simulink model "Dinamica_numerica_MPC"  (R2024b)
(part 3 of 4)

% A_drag(4,4) = (B_c*mu*rho*(cos(u_c - atan2(e_yc, e_xc) + (13*sin(3*u_c - 3*atan2(e_yc, e_xc))*(e_xc^2 + e_yc^2)^(3/2))/12 + sin(u_c - atan2(e_yc, e_xc))*(2*(e_xc^2 + e_yc^2)^(1/2) - (e_xc^2 + e_yc^2)^(3/2)/4) + sin(2*u_c - 2*atan2(e_yc, e_xc))*((5*e_xc^2)/4 + (5*e_yc^2)/4)) + (e_xc^2 + e_yc^2)^(1/2))*(delta_B + 1)*(2*cos(u_c - atan2(e_yc, e_xc) + (13*sin(3*u_c - 3*atan2(e_yc, e_xc))*(e_xc^2 + e_yc^2)^(3/2))/12 + sin(u_c - atan2(e_yc, e_xc))*(2*(e_xc^2 + e_yc^2)^(1/2) - (e_xc^2 + e_yc^2)^(3/2)/4) + sin(2*u_c - 2*atan2(e_yc, e_xc))*((5*e_xc^2)/4 + (5*e_yc^2)/4))*(e_xc^2 + e_yc^2)^(1/2) + e_xc^2 + e_yc^2 + 1)^(1/2))/(a_c*(e_xc^2 + e_yc^2)^(1/2)*(-mu/(a_c*(e_xc^2 + e_yc^2 - 1)))^(1/2)*(e_xc^2 + e_yc^2 - 1)) - (2*B_c*e_yc^2*mu*rho*(cos(u_c - atan2(e_yc, e_xc) + (13*sin(3*u_c - 3*atan2(e_yc, e_xc))*(e_xc^2 + e_yc^2)^(3/2))/12 + sin(u_c - atan2(e_yc, e_xc))*(2*(e_xc^2 + e_yc^2)^(1/2) - (e_xc^2 + e_yc^2)^(3/2)/4) + sin(2*u_c - 2*atan2(e_yc, e_xc))*((5*e_xc^2)/4 + (5*e_yc^2)/4)) + (e_xc^2 + e_yc^2)^(1/2))*(delta_B + 1)*(2*cos(u_c - atan2(e_yc, e_xc) + (13*sin(3*u_c - 3*atan2(e_yc, e_xc))*(e_xc^2 + e_yc^2)^(3/2))/12 + sin(u_c - atan2(e_yc, e_xc))*(2*(e_xc^2 + e_yc^2)^(1/2) - (e_xc^2 + e_yc^2)^(3/2)/4) + sin(2*u_c - 2*atan2(e_yc, e_xc))*((5*e_xc^2)/4 + (5*e_yc^2)/4))*(e_xc^2 + e_yc^2)^(1/2) + e_xc^2 + e_yc^2 + 1)^(1/2))/(a_c*(e_xc^2 + e_yc^2)^(1/2)*(-mu/(a_c*(e_xc^2 + e_yc^2 - 1)))^(1/2)*(e_xc^2 + e_yc^2 - 1)^2) - (B_c*e_yc^2*mu*rho*(cos(u_c - atan2(e_yc, e_xc) + (13*sin(3*u_c - 3*atan2(e_yc, e_xc))*(e_xc^2 + e_yc^2)^(3/2))/12 + sin(u_c - atan2(e_yc, e_xc))*(2*(e_xc^2 + e_yc^2)^(1/2) - (e_xc^2 + e_yc^2)^(3/2)/4) + sin(2*u_c - 2*atan2(e_yc, e_xc))*((5*e_xc^2)/4 + (5*e_yc^2)/4)) + (e_xc^2 + e_yc^2)^(1/2))*(delta_B + 1)*(2*cos(u_c - atan2(e_yc, e_xc) + (13*sin(3*u_c - 3*atan2(e_yc, e_xc))*(e_xc^2 + e_yc^2)^(3/2))/12 + sin(u_c - atan2(e_yc, e_xc))*(2*(e_xc^2 + e_yc^2)^(1/2) - (e_xc^2 + e_yc^2)^(3/2)/4) + sin(2*u_c - 2*atan2(e_yc, e_xc))*((5*e_xc^2)/4 + (5*e_yc^2)/4))*(e_xc^2 + e_yc^2)^(1/2) + e_xc^2 + e_yc^2 + 1)^(1/2))/(a_c*(e_xc^2 + e_yc^2)^(3/2)*(-mu/(a_c*(e_xc^2 + e_yc^2 - 1)))^(1/2)*(e_xc^2 + e_yc^2 - 1)) + (B_c*e_yc*mu*rho*(delta_B + 1)*(e_yc/(e_xc^2 + e_yc^2)^(1/2) + sin(u_c - atan2(e_yc, e_xc) + (13*sin(3*u_c - 3*atan2(e_yc, e_xc))*(e_xc^2 + e_yc^2)^(3/2))/12 + sin(u_c - atan2(e_yc, e_xc))*(2*(e_xc^2 + e_yc^2)^(1/2) - (e_xc^2 + e_yc^2)^(3/2)/4) + sin(2*u_c - 2*atan2(e_yc, e_xc))*((5*e_xc^2)/4 + (5*e_yc^2)/4))*(e_xc/(e_xc^2 + e_yc^2) - sin(u_c - atan2(e_yc, e_xc))*((2*e_yc)/(e_xc^2 + e_yc^2)^(1/2) - (3*e_yc*(e_xc^2 + e_yc^2)^(1/2))/4) - (5*e_yc*sin(2*u_c - 2*atan2(e_yc, e_xc)))/2 + (13*e_xc*cos(3*u_c - 3*atan2(e_yc, e_xc))*(e_xc^2 + e_yc^2)^(1/2))/4 - (13*e_yc*sin(3*u_c - 3*atan2(e_yc, e_xc))*(e_xc^2 + e_yc^2)^(1/2))/4 + (e_xc*cos(u_c - atan2(e_yc, e_xc))*(2*(e_xc^2 + e_yc^2)^(1/2) - (e_xc^2 + e_yc^2)^(3/2)/4))/(e_xc^2 + e_yc^2) + (2*e_xc*cos(2*u_c - 2*atan2(e_yc, e_xc))*((5*e_xc^2)/4 + (5*e_yc^2)/4))/(e_xc^2 + e_yc^2)))*(2*cos(u_c - atan2(e_yc, e_xc) + (13*sin(3*u_c - 3*atan2(e_yc, e_xc))*(e_xc^2 + e_yc^2)^(3/2))/12 + sin(u_c - atan2(e_yc, e_xc))*(2*(e_xc^2 + e_yc^2)^(1/2) - (e_xc^2 + e_yc^2)^(3/2)/4) + sin(2*u_c - 2*atan2(e_yc, e_xc))*((5*e_xc^2)/4 + (5*e_yc^2)/4))*(e_xc^2 + e_yc^2)^(1/2) + e_xc^2 + e_yc^2 + 1)^(1/2))/(a_c*(e_xc^2 + e_yc^2)^(1/2)*(-mu/(a_c*(e_xc^2 + e_yc^2 - 1)))^(1/2)*(e_xc^2 + e_yc^2 - 1)) - (B_c*e_yc^2*mu^2*rho*(cos(u_c - atan2(e_yc, e_xc) + (13*sin(3*u_c - 3*atan2(e_yc, e_xc))*(e_xc^2 + e_yc^2)^(3/2))/12 + sin(u_c - atan2(e_yc, e_xc))*(2*(e_xc^2 + e_yc^2)^(1/2) - (e_xc^2 + e_yc^2)^(3/2)/4) + sin(2*u_c - 2*atan2(e_yc, e_xc))*((5*e_xc^2)/4 + (5*e_yc^2)/4)) + (e_xc^2 + e_yc^2)^(1/2))*(delta_B + 1)*(2*cos(u_c - atan2(e_yc, e_xc) + (13*sin(3*u_c - 3*atan2(e_yc, e_xc))*(e_xc^2 + e_yc^2)^(3/2))/12 + sin(u_c - atan2(e_yc, e_xc))*(2*(e_xc^2 + e_yc^2)^(1/2) - (e_xc^2 + e_yc^2)^(3/2)/4) + sin(2*u_c - 2*atan2(e_yc, e_xc))*((5*e_xc^2)/4 + (5*e_yc^2)/4))*(e_xc^2 + e_yc^2)^(1/2) + e_xc^2 + e_yc^2 + 1)^(1/2))/(a_c^2*(e_xc^2 + e_yc^2)^(1/2)*(-mu/(a_c*(e_xc^2 + e_yc^2 - 1)))^(3/2)*(e_xc^2 + e_yc^2 - 1)^3) - (2*B_c*e_xc*e_yc*mu*rho*sin(u_c - atan2(e_yc, e_xc) + (13*sin(3*u_c - 3*atan2(e_yc, e_xc))*(e_xc^2 + e_yc^2)^(3/2))/12 + sin(u_c - atan2(e_yc, e_xc))*(2*(e_xc^2 + e_yc^2)^(1/2) - (e_xc^2 + e_yc^2)^(3/2)/4) + sin(2*u_c - 2*atan2(e_yc, e_xc))*((5*e_xc^2)/4 + (5*e_yc^2)/4))*(delta_B + 1)*(2*cos(u_c - atan2(e_yc, e_xc) + (13*sin(3*u_c - 3*atan2(e_yc, e_xc))*(e_xc^2 + e_yc^2)^(3/2))/12 + sin(u_c - atan2(e_yc, e_xc))*(2*(e_xc^2 + e_yc^2)^(1/2) - (e_xc^2 + e_yc^2)^(3/2)/4) + sin(2*u_c - 2*atan2(e_yc, e_xc))*((5*e_xc^2)/4 + (5*e_yc^2)/4))*(e_xc^2 + e_yc^2)^(1/2) + e_xc^2 + e_yc^2 + 1)^(1/2))/(a_c*(e_xc^2 + e_yc^2)^(1/2)*(-mu/(a_c*(e_xc^2 + e_yc^2 - 1)))^(1/2)*(e_xc^2 + e_yc^2 - 1)^2) - (B_c*e_xc*e_yc*mu*rho*sin(u_c - atan2(e_yc, e_xc) + (13*sin(3*u_c - 3*atan2(e_yc, e_xc))*(e_xc^2 + e_yc^2)^(3/2))/12 + sin(u_c - atan2(e_yc, e_xc))*(2*(e_xc^2 + e_yc^2)^(1/2) - (e_xc^2 + e_yc^2)^(3/2)/4) + sin(2*u_c - 2*atan2(e_yc, e_xc))*((5*e_xc^2)/4 + (5*e_yc^2)/4))*(delta_B + 1)*(2*cos(u_c - atan2(e_yc, e_xc) + (13*sin(3*u_c - 3*atan2(e_yc, e_xc))*(e_xc^2 + e_yc^2)^(3/2))/12 + sin(u_c - atan2(e_yc, e_xc))*(2*(e_xc^2 + e_yc^2)^(1/2) - (e_xc^2 + e_yc^2)^(3/2)/4) + sin(2*u_c - 2*atan2(e_yc, e_xc))*((5*e_xc^2)/4 + (5*e_yc^2)/4))*(e_xc^2 + e_yc^2)^(1/2) + e_xc^2 + e_yc^2 + 1)^(1/2))/(a_c*(e_xc^2 + e_yc^2)^(3/2)*(-mu/(a_c*(e_xc^2 + e_yc^2 - 1)))^(1/2)*(e_xc^2 + e_yc^2 - 1)) + (B_c*e_xc*mu*rho*sin(u_c - atan2(e_yc, e_xc) + (13*sin(3*u_c - 3*atan2(e_yc, e_xc))*(e_xc^2 + e_yc^2)^(3/2))/12 + sin(u_c - atan2(e_yc, e_xc))*(2*(e_xc^2 + e_yc^2)^(1/2) - (e_xc^2 + e_yc^2)^(3/2)/4) + sin(2*u_c - 2*atan2(e_yc, e_xc))*((5*e_xc^2)/4 + (5*e_yc^2)/4))*(delta_B + 1)*(2*e_yc + (2*e_yc*cos(u_c - atan2(e_yc, e_xc) + (13*sin(3*u_c - 3*atan2(e_yc, e_xc))*(e_xc^2 + e_yc^2)^(3/2))/12 + sin(u_c - atan2(e_yc, e_xc))*(2*(e_xc^2 + e_yc^2)^(1/2) - (e_xc^2 + e_yc^2)^(3/2)/4) + sin(2*u_c - 2*atan2(e_yc, e_xc))*((5*e_xc^2)/4 + (5*e_yc^2)/4)))/(e_xc^2 + e_yc^2)^(1/2) + 2*sin(u_c - atan2(e_yc, e_xc) + (13*sin(3*u_c - 3*atan2(e_yc, e_xc))*(e_xc^2 + e_yc^2)^(3/2))/12 + sin(u_c - atan2(e_yc, e_xc))*(2*(e_xc^2 + e_yc^2)^(1/2) - (e_xc^2 + e_yc^2)^(3/2)/4) + sin(2*u_c - 2*atan2(e_yc, e_xc))*((5*e_xc^2)/4 + (5*e_yc^2)/4))*(e_xc^2 + e_yc^2)^(1/2)*(e_xc/(e_xc^2 + e_yc^2) - sin(u_c - atan2(e_yc, e_xc))*((2*e_yc)/(e_xc^2 + e_yc^2)^(1/2) - (3*e_yc*(e_xc^2 + e_yc^2)^(1/2))/4) - (5*e_yc*sin(2*u_c - 2*atan2(e_yc, e_xc)))/2 + (13*e_xc*cos(3*u_c - 3*atan2(e_yc, e_xc))*(e_xc^2 + e_yc^2)^(1/2))/4 - (13*e_yc*sin(3*u_c - 3*atan2(e_yc, e_xc))*(e_xc^2 + e_yc^2)^(1/2))/4 + (e_xc*cos(u_c - atan2(e_yc, e_xc))*(2*(e_xc^2 + e_yc^2)^(1/2) - (e_xc^2 + e_yc^2)^(3/2)/4))/(e_xc^2 + e_yc^2) + (2*e_xc*cos(2*u_c - 2*atan2(e_yc, e_xc))*((5*e_xc^2)/4 + (5*e_yc^2)/4))/(e_xc^2 + e_yc^2))))/(2*a_c*(e_xc^2 + e_yc^2)^(1/2)*(-mu/(a_c*(e_xc^2 + e_yc^2 - 1)))^(1/2)*(e_xc^2 + e_yc^2 - 1)*(2*cos(u_c - atan2(e_yc, e_xc) + (13*sin(3*u_c - 3*atan2(e_yc, e_xc))*(e_xc^2 + e_yc^2)^(3/2))/12 + sin(u_c - atan2(e_yc, e_xc))*(2*(e_xc^2 + e_yc^2)^(1/2) - (e_xc^2 + e_yc^2)^(3/2)/4) + sin(2*u_c - 2*atan2(e_yc, e_xc))*((5*e_xc^2)/4 + (5*e_yc^2)/4))*(e_xc^2 + e_yc^2)^(1/2) + e_xc^2 + e_yc^2 + 1)^(1/2)) - (B_c*e_xc*e_yc*mu^2*rho*sin(u_c - atan2(e_yc, e_xc) + (13*sin(3*u_c - 3*atan2(e_yc, e_xc))*(e_xc^2 + e_yc^2)^(3/2))/12 + sin(u_c - atan2(e_yc, e_xc))*(2*(e_xc^2 + e_yc^2)^(1/2) - (e_xc^2 + e_yc^2)^(3/2)/4) + sin(2*u_c - 2*atan2(e_yc, e_xc))*((5*e_xc^2)/4 + (5*e_yc^2)/4))*(delta_B + 1)*(2*cos(u_c - atan2(e_yc, e_xc) + (13*sin(3*u_c - 3*atan2(e_yc, e_xc))*(e_xc^2 + e_yc^2)^(3/2))/12 + sin(u_c - atan2(e_yc, e_xc))*(2*(e_xc^2 + e_yc^2)^(1/2) - (e_xc^2 + e_yc^2)^(3/2)/4) + sin(2*u_c - 2*atan2(e_yc, e_xc))*((5*e_xc^2)/4 + (5*e_yc^2)/4))*(e_xc^2 + e_yc^2)^(1/2) + e_xc^2 + e_yc^2 + 1)^(1/2))/(a_c^2*(e_xc^2 + e_yc^2)^(1/2)*(-mu/(a_c*(e_xc^2 + e_yc^2 - 1)))^(3/2)*(e_xc^2 + e_yc^2 - 1)^3) - (B_c*e_xc*mu*rho*cos(u_c - atan2(e_yc, e_xc) + (13*sin(3*u_c - 3*atan2(e_yc, e_xc))*(e_xc^2 + e_yc^2)^(3/2))/12 + sin(u_c - atan2(e_yc, e_xc))*(2*(e_xc^2 + e_yc^2)^(1/2) - (e_xc^2 + e_yc^2)^(3/2)/4) + sin(2*u_c - 2*atan2(e_yc, e_xc))*((5*e_xc^2)/4 + (5*e_yc^2)/4))*(delta_B + 1)*(2*cos(u_c - atan2(e_yc, e_xc) + (13*sin(3*u_c - 3*atan2(e_yc, e_xc))*(e_xc^2 + e_yc^2)^(3/2))/12 + sin(u_c - atan2(e_yc, e_xc))*(2*(e_xc^2 + e_yc^2)^(1/2) - (e_xc^2 + e_yc^2)^(3/2)/4) + sin(2*u_c - 2*atan2(e_yc, e_xc))*((5*e_xc^2)/4 + (5*e_yc^2)/4))*(e_xc^2 + e_yc^2)^(1/2) + e_xc^2 + e_yc^2 + 1)^(1/2)*(e_xc/(e_xc^2 + e_yc^2) - sin(u_c - atan2(e_yc, e_xc))*((2*e_yc)/(e_xc^2 + e_yc^2)^(1/2) - (3*e_yc*(e_xc^2 + e_yc^2)^(1/2))/4) - (5*e_yc*sin(2*u_c - 2*atan2(e_yc, e_xc)))/2 + (13*e_xc*cos(3*u_c - 3*atan2(e_yc, e_xc))*(e_xc^2 + e_yc^2)^(1/2))/4 - (13*e_yc*sin(3*u_c - 3*atan2(e_yc, e_xc))*(e_xc^2 + e_yc^2)^(1/2))/4 + (e_xc*cos(u_c - atan2(e_yc, e_xc))*(2*(e_xc^2 + e_yc^2)^(1/2) - (e_xc^2 + e_yc^2)^(3/2)/4))/(e_xc^2 + e_yc^2) + (2*e_xc*cos(2*u_c - 2*atan2(e_yc, e_xc))*((5*e_xc^2)/4 + (5*e_yc^2)/4))/(e_xc^2 + e_yc^2)))/(a_c*(e_xc^2 + e_yc^2)^(1/2)*(-mu/(a_c*(e_xc^2 + e_yc^2 - 1)))^(1/2)*(e_xc^2 + e_yc^2 - 1)) + (B_c*e_yc*mu*rho*(cos(u_c - atan2(e_yc, e_xc) + (13*sin(3*u_c - 3*atan2(e_yc, e_xc))*(e_xc^2 + e_yc^2)^(3/2))/12 + sin(u_c - atan2(e_yc, e_xc))*(2*(e_xc^2 + e_yc^2)^(1/2) - (e_xc^2 + e_yc^2)^(3/2)/4) + sin(2*u_c - 2*atan2(e_yc, e_xc))*((5*e_xc^2)/4 + (5*e_yc^2)/4)) + (e_xc^2 + e_yc^2)^(1/2))*(delta_B + 1)*(2*e_yc + (2*e_yc*cos(u_c - atan2(e_yc, e_xc) + (13*sin(3*u_c - 3*atan2(e_yc, e_xc))*(e_xc^2 + e_yc^2)^(3/2))/12 + sin(u_c - atan2(e_yc, e_xc))*(2*(e_xc^2 + e_yc^2)^(1/2) - (e_xc^2 + e_yc^2)^(3/2)/4) + sin(2*u_c - 2*atan2(e_yc, e_xc))*((5*e_xc^2)/4 + (5*e_yc^2)/4)))/(e_xc^2 + e_yc^2)^(1/2) + 2*sin(u_c - atan2(e_yc, e_xc) + (13*sin(3*u_c - 3*atan2(e_yc, e_xc))*(e_xc^2 + e_yc^2)^(3/2))/12 + sin(u_c - atan2(e_yc, e_xc))*(2*(e_xc^2 + e_yc^2)^(1/2) - (e_xc^2 + e_yc^2)^(3/2)/4) + sin(2*u_c - 2*atan2(e_yc, e_xc))*((5*e_xc^2)/4 + (5*e_yc^2)/4))*(e_xc^2 + e_yc^2)^(1/2)*(e_xc/(e_xc^2 + e_yc^2) - sin(u_c - atan2(e_yc, e_xc))*((2*e_yc)/(e_xc^2 + e_yc^2)^(1/2) - (3*e_yc*(e_xc^2 + e_yc^2)^(1/2))/4) - (5*e_yc*sin(2*u_c - 2*atan2(e_yc, e_xc)))/2 + (13*e_xc*cos(3*u_c - 3*atan2(e_yc, e_xc))*(e_xc^2 + e_yc^2)^(1/2))/4 - (13*e_yc*sin(3*u_c - 3*atan2(e_yc, e_xc))*(e_xc^2 + e_yc^2)^(1/2))/4 + (e_xc*cos(u_c - atan2(e_yc, e_xc))*(2*(e_xc^2 + e_yc^2)^(1/2) - (e_xc^2 + e_yc^2)^(3/2)/4))/(e_xc^2 + e_yc^2) + (2*e_xc*cos(2*u_c - 2*atan2(e_yc, e_xc))*((5*e_xc^2)/4 + (5*e_yc^2)/4))/(e_xc^2 + e_yc^2))))/(2*a_c*(e_xc^2 + e_yc^2)^(1/2)*(-mu/(a_c*(e_xc^2 + e_yc^2 - 1)))^(1/2)*(e_xc^2 + e_yc^2 - 1)*(2*cos(u_c - atan2(e_yc, e_xc) + (13*sin(3*u_c - 3*atan2(e_yc, e_xc))*(e_xc^2 + e_yc^2)^(3/2))/12 + sin(u_c - atan2(e_yc, e_xc))*(2*(e_xc^2 + e_yc^2)^(1/2) - (e_xc^2 + e_yc^2)^(3/2)/4) + sin(2*u_c - 2*atan2(e_yc, e_xc))*((5*e_xc^2)/4 + (5*e_yc^2)/4))*(e_xc^2 + e_yc^2)^(1/2) + e_xc^2 + e_yc^2 + 1)^(1/2));
% A_drag(4,5) = 0;
% A_drag(4,6) = (B_c*e_xc*mu*rho*sin(u_c - atan2(e_yc, e_xc) + (13*sin(3*u_c - 3*atan2(e_yc, e_xc))*(e_xc^2 + e_yc^2)^(3/2))/12 + sin(u_c - atan2(e_yc, e_xc))*(2*(e_xc^2 + e_yc^2)^(1/2) - (e_xc^2 + e_yc^2)^(3/2)/4) + sin(2*u_c - 2*atan2(e_yc, e_xc))*((5*e_xc^2)/4 + (5*e_yc^2)/4))^2*(delta_B + 1)*(1/tan(i_c) + (2*cos(2*u_c - 2*atan2(e_yc, e_xc))*((5*e_xc^2)/4 + (5*e_yc^2)/4))/tan(i_c) + (13*cos(3*u_c - 3*atan2(e_yc, e_xc))*(e_xc^2 + e_yc^2)^(3/2))/(4*tan(i_c)) + (cos(u_c - atan2(e_yc, e_xc))*(2*(e_xc^2 + e_yc^2)^(1/2) - (e_xc^2 + e_yc^2)^(3/2)/4))/tan(i_c)))/(a_c*(-mu/(a_c*(e_xc^2 + e_yc^2 - 1)))^(1/2)*(e_xc^2 + e_yc^2 - 1)*(2*cos(u_c - atan2(e_yc, e_xc) + (13*sin(3*u_c - 3*atan2(e_yc, e_xc))*(e_xc^2 + e_yc^2)^(3/2))/12 + sin(u_c - atan2(e_yc, e_xc))*(2*(e_xc^2 + e_yc^2)^(1/2) - (e_xc^2 + e_yc^2)^(3/2)/4) + sin(2*u_c - 2*atan2(e_yc, e_xc))*((5*e_xc^2)/4 + (5*e_yc^2)/4))*(e_xc^2 + e_yc^2)^(1/2) + e_xc^2 + e_yc^2 + 1)^(1/2)) + (B_c*e_yc*mu*rho*sin(u_c - atan2(e_yc, e_xc) + (13*sin(3*u_c - 3*atan2(e_yc, e_xc))*(e_xc^2 + e_yc^2)^(3/2))/12 + sin(u_c - atan2(e_yc, e_xc))*(2*(e_xc^2 + e_yc^2)^(1/2) - (e_xc^2 + e_yc^2)^(3/2)/4) + sin(2*u_c - 2*atan2(e_yc, e_xc))*((5*e_xc^2)/4 + (5*e_yc^2)/4))*(cos(u_c - atan2(e_yc, e_xc) + (13*sin(3*u_c - 3*atan2(e_yc, e_xc))*(e_xc^2 + e_yc^2)^(3/2))/12 + sin(u_c - atan2(e_yc, e_xc))*(2*(e_xc^2 + e_yc^2)^(1/2) - (e_xc^2 + e_yc^2)^(3/2)/4) + sin(2*u_c - 2*atan2(e_yc, e_xc))*((5*e_xc^2)/4 + (5*e_yc^2)/4)) + (e_xc^2 + e_yc^2)^(1/2))*(delta_B + 1)*(1/tan(i_c) + (2*cos(2*u_c - 2*atan2(e_yc, e_xc))*((5*e_xc^2)/4 + (5*e_yc^2)/4))/tan(i_c) + (13*cos(3*u_c - 3*atan2(e_yc, e_xc))*(e_xc^2 + e_yc^2)^(3/2))/(4*tan(i_c)) + (cos(u_c - atan2(e_yc, e_xc))*(2*(e_xc^2 + e_yc^2)^(1/2) - (e_xc^2 + e_yc^2)^(3/2)/4))/tan(i_c)))/(a_c*(-mu/(a_c*(e_xc^2 + e_yc^2 - 1)))^(1/2)*(e_xc^2 + e_yc^2 - 1)*(2*cos(u_c - atan2(e_yc, e_xc) + (13*sin(3*u_c - 3*atan2(e_yc, e_xc))*(e_xc^2 + e_yc^2)^(3/2))/12 + sin(u_c - atan2(e_yc, e_xc))*(2*(e_xc^2 + e_yc^2)^(1/2) - (e_xc^2 + e_yc^2)^(3/2)/4) + sin(2*u_c - 2*atan2(e_yc, e_xc))*((5*e_xc^2)/4 + (5*e_yc^2)/4))*(e_xc^2 + e_yc^2)^(1/2) + e_xc^2 + e_yc^2 + 1)^(1/2)) - (B_c*e_xc*mu*rho*cos(u_c - atan2(e_yc, e_xc) + (13*sin(3*u_c - 3*atan2(e_yc, e_xc))*(e_xc^2 + e_yc^2)^(3/2))/12 + sin(u_c - atan2(e_yc, e_xc))*(2*(e_xc^2 + e_yc^2)^(1/2) - (e_xc^2 + e_yc^2)^(3/2)/4) + sin(2*u_c - 2*atan2(e_yc, e_xc))*((5*e_xc^2)/4 + (5*e_yc^2)/4))*(delta_B + 1)*(2*cos(u_c - atan2(e_yc, e_xc) + (13*sin(3*u_c - 3*atan2(e_yc, e_xc))*(e_xc^2 + e_yc^2)^(3/2))/12 + sin(u_c - atan2(e_yc, e_xc))*(2*(e_xc^2 + e_yc^2)^(1/2) - (e_xc^2 + e_yc^2)^(3/2)/4) + sin(2*u_c - 2*atan2(e_yc, e_xc))*((5*e_xc^2)/4 + (5*e_yc^2)/4))*(e_xc^2 + e_yc^2)^(1/2) + e_xc^2 + e_yc^2 + 1)^(1/2)*(1/tan(i_c) + (2*cos(2*u_c - 2*atan2(e_yc, e_xc))*((5*e_xc^2)/4 + (5*e_yc^2)/4))/tan(i_c) + (13*cos(3*u_c - 3*atan2(e_yc, e_xc))*(e_xc^2 + e_yc^2)^(3/2))/(4*tan(i_c)) + (cos(u_c - atan2(e_yc, e_xc))*(2*(e_xc^2 + e_yc^2)^(1/2) - (e_xc^2 + e_yc^2)^(3/2)/4))/tan(i_c)))/(a_c*(e_xc^2 + e_yc^2)^(1/2)*(-mu/(a_c*(e_xc^2 + e_yc^2 - 1)))^(1/2)*(e_xc^2 + e_yc^2 - 1)) + (B_c*e_yc*mu*rho*sin(u_c - atan2(e_yc, e_xc) + (13*sin(3*u_c - 3*atan2(e_yc, e_xc))*(e_xc^2 + e_yc^2)^(3/2))/12 + sin(u_c - atan2(e_yc, e_xc))*(2*(e_xc^2 + e_yc^2)^(1/2) - (e_xc^2 + e_yc^2)^(3/2)/4) + sin(2*u_c - 2*atan2(e_yc, e_xc))*((5*e_xc^2)/4 + (5*e_yc^2)/4))*(delta_B + 1)*(2*cos(u_c - atan2(e_yc, e_xc) + (13*sin(3*u_c - 3*atan2(e_yc, e_xc))*(e_xc^2 + e_yc^2)^(3/2))/12 + sin(u_c - atan2(e_yc, e_xc))*(2*(e_xc^2 + e_yc^2)^(1/2) - (e_xc^2 + e_yc^2)^(3/2)/4) + sin(2*u_c - 2*atan2(e_yc, e_xc))*((5*e_xc^2)/4 + (5*e_yc^2)/4))*(e_xc^2 + e_yc^2)^(1/2) + e_xc^2 + e_yc^2 + 1)^(1/2)*(1/tan(i_c) + (2*cos(2*u_c - 2*atan2(e_yc, e_xc))*((5*e_xc^2)/4 + (5*e_yc^2)/4))/tan(i_c) + (13*cos(3*u_c - 3*atan2(e_yc, e_xc))*(e_xc^2 + e_yc^2)^(3/2))/(4*tan(i_c)) + (cos(u_c - atan2(e_yc, e_xc))*(2*(e_xc^2 + e_yc^2)^(1/2) - (e_xc^2 + e_yc^2)^(3/2)/4))/tan(i_c)))/(a_c*(e_xc^2 + e_yc^2)^(1/2)*(-mu/(a_c*(e_xc^2 + e_yc^2 - 1)))^(1/2)*(e_xc^2 + e_yc^2 - 1));
% A_drag(4,7) = (B_c*e_yc*mu*rho*(cos(u_c - atan2(e_yc, e_xc) + (13*sin(3*u_c - 3*atan2(e_yc, e_xc))*(e_xc^2 + e_yc^2)^(3/2))/12 + sin(u_c - atan2(e_yc, e_xc))*(2*(e_xc^2 + e_yc^2)^(1/2) - (e_xc^2 + e_yc^2)^(3/2)/4) + sin(2*u_c - 2*atan2(e_yc, e_xc))*((5*e_xc^2)/4 + (5*e_yc^2)/4)) + (e_xc^2 + e_yc^2)^(1/2))*(2*cos(u_c - atan2(e_yc, e_xc) + (13*sin(3*u_c - 3*atan2(e_yc, e_xc))*(e_xc^2 + e_yc^2)^(3/2))/12 + sin(u_c - atan2(e_yc, e_xc))*(2*(e_xc^2 + e_yc^2)^(1/2) - (e_xc^2 + e_yc^2)^(3/2)/4) + sin(2*u_c - 2*atan2(e_yc, e_xc))*((5*e_xc^2)/4 + (5*e_yc^2)/4))*(e_xc^2 + e_yc^2)^(1/2) + e_xc^2 + e_yc^2 + 1)^(1/2))/(a_c*(e_xc^2 + e_yc^2)^(1/2)*(-mu/(a_c*(e_xc^2 + e_yc^2 - 1)))^(1/2)*(e_xc^2 + e_yc^2 - 1)) + (B_c*e_xc*mu*rho*sin(u_c - atan2(e_yc, e_xc) + (13*sin(3*u_c - 3*atan2(e_yc, e_xc))*(e_xc^2 + e_yc^2)^(3/2))/12 + sin(u_c - atan2(e_yc, e_xc))*(2*(e_xc^2 + e_yc^2)^(1/2) - (e_xc^2 + e_yc^2)^(3/2)/4) + sin(2*u_c - 2*atan2(e_yc, e_xc))*((5*e_xc^2)/4 + (5*e_yc^2)/4))*(2*cos(u_c - atan2(e_yc, e_xc) + (13*sin(3*u_c - 3*atan2(e_yc, e_xc))*(e_xc^2 + e_yc^2)^(3/2))/12 + sin(u_c - atan2(e_yc, e_xc))*(2*(e_xc^2 + e_yc^2)^(1/2) - (e_xc^2 + e_yc^2)^(3/2)/4) + sin(2*u_c - 2*atan2(e_yc, e_xc))*((5*e_xc^2)/4 + (5*e_yc^2)/4))*(e_xc^2 + e_yc^2)^(1/2) + e_xc^2 + e_yc^2 + 1)^(1/2))/(a_c*(e_xc^2 + e_yc^2)^(1/2)*(-mu/(a_c*(e_xc^2 + e_yc^2 - 1)))^(1/2)*(e_xc^2 + e_yc^2 - 1));
% A_drag(5,1) = 0;
% A_drag(5,2) = 0;
% A_drag(5,3) = 0;
% A_drag(5,4) = 0;
% A_drag(5,5) = 0;
% A_drag(5,6) = 0;
% A_drag(5,7) = 0;
% A_drag(6,1) = 0;
% A_drag(6,2) = 0;
% A_drag(6,3) = 0;
% A_drag(6,4) = 0;
% A_drag(6,5) = 0;
% A_drag(6,6) = 0;
% A_drag(6,7) = 0;
% A_drag(7,1) = 0;
% A_drag(7,2) = 0;
% A_drag(7,3) = 0;
% A_drag(7,4) = 0;
% A_drag(7,5) = 0;
% A_drag(7,6) = 0;
% A_drag(7,7) = 0;

%----------------------------------------------------------------------------




% Total matrix plant:
% A_J2
% A_drag

A = A_kep + A_J2 + A_drag;


% Control Matrix


% B   = [2/eta*e_c*sin(nu_c),      2/eta*(1+e_c*cos(nu_c)),   0;
%     -2*eta^2/(1+e_c*cos(nu_c)),                  0,   0;
%     eta*sin(u_c),   eta*((2+e_c*cos(nu_c))*cos(u_c)+e_xc)/(1+e_c*cos(nu_c)),      eta*e_yc*sin(u_c)/tan(i_c)/(1+e_c*cos(nu_c));
%     -eta*cos(u_c),   eta*((2+e_c*cos(nu_c))*sin(u_c)+e_yc)/(1+e_c*cos(nu_c)),     -eta*e_xc*sin(u_c)/tan(i_c)/(1+e_c*cos(nu_c));
%     0            0,       eta*cos(u_c)/(1+e_c*cos(nu_c))
%     0            0,       eta*sin(u_c)/(1+e_c*cos(nu_c)); 
%     zeros(1,3)].*1/(a_c*n_c);

theta_c = nu_c + om_c; % true argument of latitude
B   = [2/eta*e_c*sin(nu_c),      2/eta*(1+e_c*cos(nu_c)),   0;
    -2*eta^2/(1+e_c*cos(nu_c)),                  0,   0;
    eta*sin(theta_c),   eta*((2+e_c*cos(nu_c))*cos(theta_c)+e_xc)/(1+e_c*cos(nu_c)),      eta*e_yc*sin(theta_c)/tan(i_c)/(1+e_c*cos(nu_c));
    -eta*cos(theta_c),   eta*((2+e_c*cos(nu_c))*sin(theta_c)+e_yc)/(1+e_c*cos(nu_c)),     -eta*e_xc*sin(theta_c)/tan(i_c)/(1+e_c*cos(nu_c));
    0            0,       eta*cos(theta_c)/(1+e_c*cos(nu_c))
    0            0,       eta*sin(theta_c)/(1+e_c*cos(nu_c)); 
    zeros(1,3)].*1/(a_c*n_c);




end
